simulink model "RWLNN_2m__"  (R2015b)
settings: Solver=ode1  StartTime=0.0  StopTime=t_sim  FixedStep=t_prob  RelTol=1e-3
values from neighbouring files (symbols this model uses):
  ksi = 1    [RWLNN_weights (2).mat]
  lr = 0.01    [RWLNN_weights (2).mat]
  lra = 0.001    [RWLNN_weights (2).mat]
  lrb = 0.001    [RWLNN_weights (2).mat]
  lrin = 0.001    [RWLNN_weights (2).mat]
  T1 = 0.203    [RWLNN_weights (2).mat]
  T2 = 0.203    [RWLNN_weights (2).mat]
  Tc = 0.0012    [RWLNN_weights (2).mat]
  w0 = 40    [RWLNN_weights (2).mat]
  w_init = [0.41  0  0.42; 0  0  -0.04]    [RWLNN_weights (2).mat]
  w_out_init = [-5 0 5]    [RWLNN_weights (2).mat]
undefined symbols (not defined in the file or in its folder): Lz
libraries: neural x3, simulink x1
settings Model: Creator=mateuszzychlewicz  LastModifiedBy=mateuszzychlewicz
settings DataIOCC: LimitDataPoints=off  SaveFormat=Array  TimeSaveName=t  OutputSaveName=y
settings OptimizationCC: EfficientMapNaN2IntZero=off
settings HardwareCC: TargetBitPerLong=64  TargetBitPerPointer=64  TargetLongLongMode=on  TargetIntDivRoundTo=Zero  TargetEndianess=LittleEndian  TargetWordSize=64  TargetHWDeviceType=MATLAB Host  ProdEqTarget=off
settings CodeAppCC: MaxIdLength=128
settings GRTTargetCC: CombineOutputUpdateFcns=off  GRTInterface=on

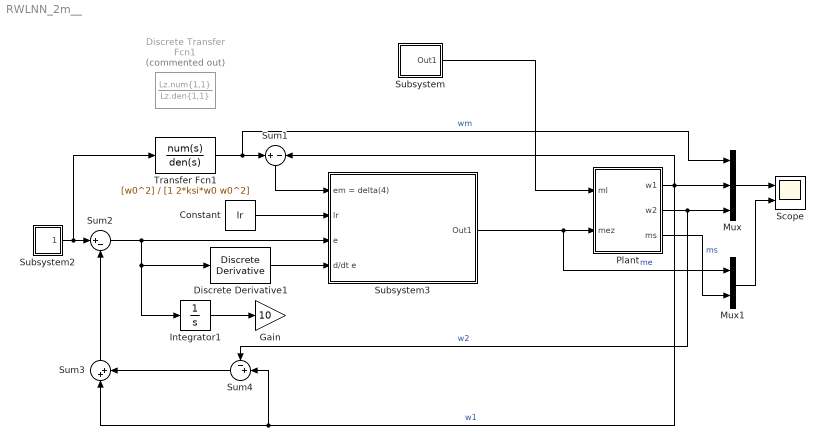
== system RWLNN_2m__ ==
  Constant : Constant  Value=lr
  Discrete Transfer Fcn1 : DiscreteTransferFcn  Commented=on  Numerator=Lz.num{1,1}  Denominator=Lz.den{1,1}
  Discrete Derivative1 : simulink/Discrete/Discrete Derivative  gainval=0.001  ICPrevScaledInput=0.0  InputProcessing=Inherited  OutMin=[]  OutMax=[]  OutDataType=fixdt(1, 16)  OutScaling=2^-10  DoSatur=off
  Gain : Gain  Gain=10
  Integrator1 : Integrator
  Mux : Mux  Inputs=3
  Mux1 : Mux  Inputs=2
  Plant : Subsystem
  Scope : Scope  NumInputPorts=2
  Subsystem : Subsystem
  Subsystem2 : Subsystem
      mask Display: disp('w_{ref}', 'texmode', 'on')
  Subsystem3 : Subsystem
  Sum1 : Sum  Inputs=+-
  Sum2 : Sum  Inputs=|+-
  Sum3 : Sum  Inputs=|++
  Sum4 : Sum  Inputs=-+|
  Transfer Fcn1 : TransferFcn  Numerator=[w0^2]  Denominator=[1 2*ksi*w0 w0^2]
  wires:
  Subsystem2/1(Out1) -> Transfer Fcn1/1, Sum2/1
  Plant/1(w1) -> Sum3/1, Sum4/2, Mux/2, Sum1/2  "w1"
  Sum2/1 -> Discrete Derivative1/1, Integrator1/1, Subsystem3/3(e)
  Transfer Fcn1/1 -> Mux/1, Sum1/1  "wm"
  Sum1/1 -> Subsystem3/1(em = delta(4))
  Plant/2(w2) -> Sum4/1, Mux/3  "w2"
  Mux/1 -> Scope/1
  Plant/3(ms) -> Mux1/2  "ms"
  Mux1/1 -> Scope/2
  Constant/1 -> Subsystem3/2(lr)
  Subsystem/1(Out1) -> Plant/1(ml)
  Integrator1/1 -> Gain/1
  Sum3/1 -> Sum2/2
  Discrete Derivative1/1 -> Subsystem3/4(d/dt e)
  Subsystem3/1(Out1) -> Mux1/1, Plant/2(mez)  "me"
  Sum4/1 -> Sum3/2

== system RWLNN_2m__/Plant ==
  ml : Inport
  mez : Inport  Port=2
  Sum3 : Sum  Inputs=-+|
  Sum4 : Sum  Inputs=-+|
  Sum5 : Sum  Inputs=|+-
  Transfer Fcn1 : TransferFcn  Denominator=[Tc 0]
  Transfer Fcn3 : TransferFcn  Denominator=[T1 0]
  Transfer Fcn4 : TransferFcn  Denominator=[1.5*T2 0]
  w1 : Outport
  w2 : Outport  Port=2
  ms : Outport  Port=3
  wires:
  Sum3/1 -> Transfer Fcn3/1
  mez/1 -> Sum3/2
  ml/1 -> Sum4/1
  Transfer Fcn3/1 -> w1/1, Sum5/1
  Transfer Fcn4/1 -> w2/1, Sum5/2
  Transfer Fcn1/1 -> ms/1, Sum3/1, Sum4/2
  Sum4/1 -> Transfer Fcn4/1
  Sum5/1 -> Transfer Fcn1/1

== system RWLNN_2m__/Subsystem ==
  Step : Step  Time=9  SampleTime=0
  Step1 : Step  Time=11  SampleTime=0
  Sum5 : Sum  Inputs=+-
  Out1 : Outport
  wires:
  Sum5/1 -> Out1/1
  Step/1 -> Sum5/1
  Step1/1 -> Sum5/2

== system RWLNN_2m__/Subsystem2 ==
  Gain : Gain
  Manual Switch : ManualSwitch
  Pulse Generator : DiscretePulseGenerator  PulseType=Time based  Amplitude=0.25  Period=5  PulseWidth=50  PhaseDelay=1
  Pulse Generator1 : DiscretePulseGenerator  PulseType=Time based  Amplitude=0.25  Period=5  PulseWidth=50  PhaseDelay=3.5
  Signal Generator : SignalGenerator  WaveForm=square  Amplitude=0.25  Frequency=0.2
  Sum5 : Sum  Inputs=+-
  Transfer Fcn2 : TransferFcn  Denominator=[0.03 1]
  Out1 : Outport
  wires:
  Sum5/1 -> Manual Switch/2
  Pulse Generator/1 -> Sum5/1
  Pulse Generator1/1 -> Sum5/2
  Signal Generator/1 -> Gain/1
  Gain/1 -> Manual Switch/1
  Manual Switch/1 -> Transfer Fcn2/1
  Transfer Fcn2/1 -> Out1/1

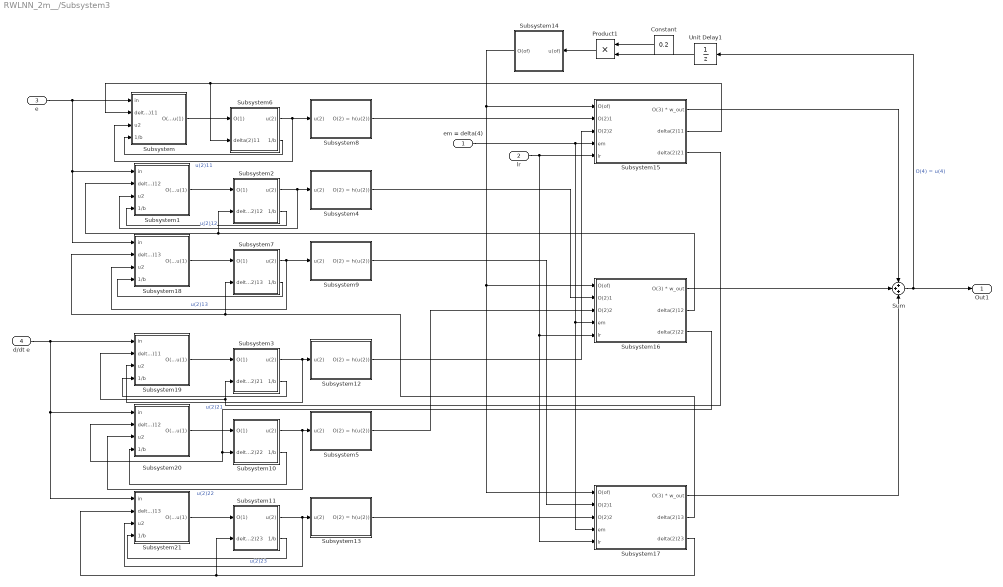
== system RWLNN_2m__/Subsystem3 ==
  em = delta(4) : Inport
  lr : Inport  Port=2
  e : Inport  Port=3
  d/dt e : Inport  Port=4
  Constant : Constant  Value=0.2
  Product1 : Product
  Subsystem : Subsystem
  Subsystem1 : Subsystem
  Subsystem10 : Subsystem
  Subsystem11 : Subsystem
  Subsystem12 : Subsystem
  Subsystem13 : Subsystem
  Subsystem14 : Subsystem
  Subsystem15 : Subsystem
  Subsystem16 : Subsystem
  Subsystem17 : Subsystem
  Subsystem18 : Subsystem
  Subsystem19 : Subsystem
  Subsystem2 : Subsystem
  Subsystem20 : Subsystem
  Subsystem21 : Subsystem
  Subsystem3 : Subsystem
  Subsystem4 : Subsystem
  Subsystem5 : Subsystem
  Subsystem6 : Subsystem
  Subsystem7 : Subsystem
  Subsystem8 : Subsystem
  Subsystem9 : Subsystem
  Sum : Sum  Inputs=+++
  Unit Delay1 : UnitDelay  SampleTime=-1
  Out1 : Outport
  wires:
  Constant/1 -> Product1/1
  Subsystem11/2(1/b) -> Subsystem21/4(1/b)
  Subsystem10/2(1/b) -> Subsystem20/4(1/b)
  Subsystem3/2(1/b) -> Subsystem19/4(1/b)
  d/dt e/1 -> Subsystem19/1(in), Subsystem20/1(in), Subsystem21/1(in)
  Subsystem21/1(O(1) = u(1)) -> Subsystem11/1(O(1))
  Subsystem20/1(O(1) = u(1)) -> Subsystem10/1(O(1))
  Subsystem19/1(O(1) = u(1)) -> Subsystem3/1(O(1))
  Subsystem7/2(1/b) -> Subsystem18/4(1/b)
  Subsystem2/2(1/b) -> Subsystem1/4(1/b)
  Subsystem6/2(1/b) -> Subsystem/4(1/b)
  Subsystem18/1(O(1) = u(1)) -> Subsystem7/1(O(1))
  Subsystem1/1(O(1) = u(1)) -> Subsystem2/1(O(1))
  Subsystem/1(O(1) = u(1)) -> Subsystem6/1(O(1))
  Subsystem17/3(delta(2)23) -> Subsystem11/2(delta(2)23), Subsystem21/2(delta(2)13)
  Subsystem16/3(delta(2)22) -> Subsystem10/2(delta(2)22), Subsystem20/2(delta(2)12)
  Subsystem15/3(delta(2)21) -> Subsystem19/2(delta(2)11), Subsystem3/2(delta(2)21)
  Subsystem17/2(delta(2)13) -> Subsystem18/2(delta(2)13), Subsystem7/2(delta(2)13)
  Subsystem16/2(delta(2)12) -> Subsystem1/2(delta(2)12), Subsystem2/2(delta(2)12)
  Subsystem4/1(O(2) = h(u(2))) -> Subsystem16/2(O(2)1)
  Subsystem5/1(O(2) = h(u(2))) -> Subsystem16/3(O(2)2)
  Subsystem8/1(O(2) = h(u(2))) -> Subsystem15/2(O(2)1)
  Subsystem13/1(O(2) = h(u(2))) -> Subsystem17/3(O(2)2)
  Subsystem12/1(O(2) = h(u(2))) -> Subsystem15/3(O(2)2)
  Subsystem9/1(O(2) = h(u(2))) -> Subsystem17/2(O(2)1)
  Sum/1 -> Unit Delay1/1, Out1/1  "O(4) = u(4)"
  Subsystem15/2(delta(2)11) -> Subsystem6/2(delta(2)11), Subsystem/2(delta(2)11)
  lr/1 -> Subsystem15/5(lr), Subsystem16/5(lr), Subsystem17/5(lr)
  Product1/1 -> Subsystem14/1(u(of))
  Unit Delay1/1 -> Product1/2
  Subsystem7/1(u(2)) -> Subsystem9/1(u(2)), Subsystem18/3(u2)  "u(2)13"
  Subsystem11/1(u(2)) -> Subsystem13/1(u(2)), Subsystem21/3(u2)  "u(2)23"
  Subsystem10/1(u(2)) -> Subsystem5/1(u(2)), Subsystem20/3(u2)  "u(2)22"
  Subsystem3/1(u(2)) -> Subsystem12/1(u(2)), Subsystem19/3(u2)  "u(2)21"
  Subsystem14/1(O(of)) -> Subsystem15/1(O(of)), Subsystem16/1(O(of)), Subsystem17/1(O(of))
  em = delta(4)/1 -> Subsystem15/4(em), Subsystem16/4(em), Subsystem17/4(em)
  Subsystem15/1(O(3) * w_out) -> Sum/1
  e/1 -> Subsystem/1(in), Subsystem1/1(in), Subsystem18/1(in)
  Subsystem2/1(u(2)) -> Subsystem4/1(u(2)), Subsystem1/3(u2)  "u(2)12"
  Subsystem6/1(u(2)) -> Subsystem8/1(u(2)), Subsystem/3(u2)  "u(2)11"
  Subsystem17/1(O(3) * w_out) -> Sum/3
  Subsystem16/1(O(3) * w_out) -> Sum/2

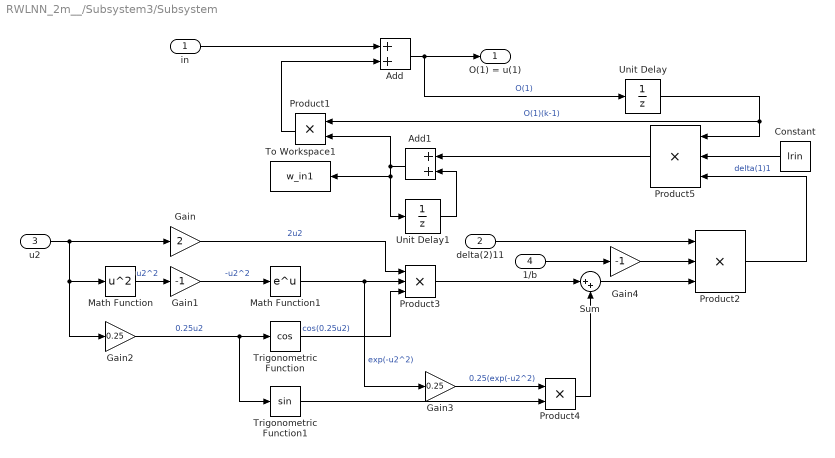
== system RWLNN_2m__/Subsystem3/Subsystem ==
  in : Inport
  delta(2)11 : Inport  Port=2
  u2 : Inport  Port=3
  1/b : Inport  Port=4
  Add : Sum
  Add1 : Sum
  Constant : Constant  Value=lrin
  Gain : Gain  Gain=2
  Gain1 : Gain  Gain=-1
  Gain2 : Gain  Gain=0.25
  Gain3 : Gain  Gain=0.25
  Gain4 : Gain  Gain=-1
  Math Function : Math  Operator=square  SaturateOnIntegerOverflow=on
  Math Function1 : Math  SaturateOnIntegerOverflow=on
  Product1 : Product
  Product2 : Product  Inputs=3
  Product3 : Product  Inputs=3
  Product4 : Product
  Product5 : Product  Inputs=3
  Sum : Sum  Inputs=|++
  To Workspace1 : ToWorkspace  VariableName=w_in1  SampleTime=-1
  Trigonometric Function : Trigonometry  Operator=cos
  Trigonometric Function1 : Trigonometry
  Unit Delay : UnitDelay  SampleTime=-1
  Unit Delay1 : UnitDelay  InitialCondition=w_init(1)  SampleTime=-1
  O(1) = u(1) : Outport
  wires:
  Product1/1 -> Add/2
  Unit Delay1/1 -> Add1/2
  Add1/1 -> Product1/2, Unit Delay1/1, To Workspace1/1
  Product5/1 -> Add1/1
  Constant/1 -> Product5/2
  Product2/1 -> Product5/3  "delta(1)1"
  1/b/1 -> Gain4/1
  Gain4/1 -> Product2/2
  Sum/1 -> Product2/3
  Product4/1 -> Sum/2
  Trigonometric Function1/1 -> Product4/2
  Gain3/1 -> Product4/1  "0.25(exp(-u2^2)"
  Product3/1 -> Sum/1
  Trigonometric Function/1 -> Product3/3  "cos(0.25u2)"
  Gain2/1 -> Trigonometric Function/1, Trigonometric Function1/1  "0.25u2"
  Math Function1/1 -> Product3/2, Gain3/1  "exp(-u2^2)"
  Gain1/1 -> Math Function1/1  "-u2^2"
  Math Function/1 -> Gain1/1  "u2^2"
  Gain/1 -> Product3/1  "2u2"
  u2/1 -> Gain/1, Math Function/1, Gain2/1
  delta(2)11/1 -> Product2/1
  Unit Delay/1 -> Product5/1, Product1/1  "O(1)(k-1)"
  in/1 -> Add/1
  Add/1 -> O(1) = u(1)/1, Unit Delay/1  "O(1)"

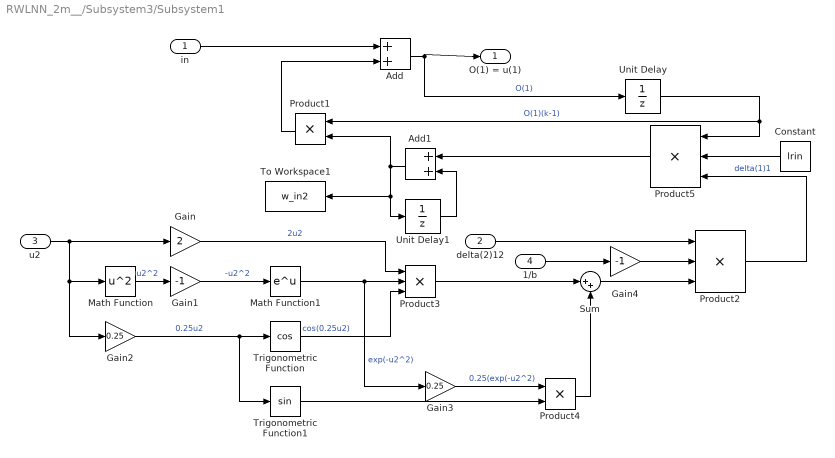
== system RWLNN_2m__/Subsystem3/Subsystem1 ==
  in : Inport
  delta(2)12 : Inport  Port=2
  u2 : Inport  Port=3
  1/b : Inport  Port=4
  Add : Sum
  Add1 : Sum
  Constant : Constant  Value=lrin
  Gain : Gain  Gain=2
  Gain1 : Gain  Gain=-1
  Gain2 : Gain  Gain=0.25
  Gain3 : Gain  Gain=0.25
  Gain4 : Gain  Gain=-1
  Math Function : Math  Operator=square  SaturateOnIntegerOverflow=on
  Math Function1 : Math  SaturateOnIntegerOverflow=on
  Product1 : Product
  Product2 : Product  Inputs=3
  Product3 : Product  Inputs=3
  Product4 : Product
  Product5 : Product  Inputs=3
  Sum : Sum  Inputs=|++
  To Workspace1 : ToWorkspace  VariableName=w_in2  SampleTime=-1
  Trigonometric Function : Trigonometry  Operator=cos
  Trigonometric Function1 : Trigonometry
  Unit Delay : UnitDelay  SampleTime=-1
  Unit Delay1 : UnitDelay  InitialCondition=w_init(2)  SampleTime=-1
  O(1) = u(1) : Outport
  wires:
  Add1/1 -> Unit Delay1/1, To Workspace1/1, Product1/2
  Add/1 -> Unit Delay/1, O(1) = u(1)/1  "O(1)"
  in/1 -> Add/1
  Unit Delay/1 -> Product1/1, Product5/1  "O(1)(k-1)"
  delta(2)12/1 -> Product2/1
  u2/1 -> Gain2/1, Math Function/1, Gain/1
  Gain/1 -> Product3/1  "2u2"
  Math Function/1 -> Gain1/1  "u2^2"
  Gain1/1 -> Math Function1/1  "-u2^2"
  Math Function1/1 -> Gain3/1, Product3/2  "exp(-u2^2)"
  Gain2/1 -> Trigonometric Function1/1, Trigonometric Function/1  "0.25u2"
  Trigonometric Function/1 -> Product3/3  "cos(0.25u2)"
  Product3/1 -> Sum/1
  Gain3/1 -> Product4/1  "0.25(exp(-u2^2)"
  Trigonometric Function1/1 -> Product4/2
  Product4/1 -> Sum/2
  Sum/1 -> Product2/3
  Gain4/1 -> Product2/2
  1/b/1 -> Gain4/1
  Product2/1 -> Product5/3  "delta(1)1"
  Constant/1 -> Product5/2
  Product5/1 -> Add1/1
  Unit Delay1/1 -> Add1/2
  Product1/1 -> Add/2

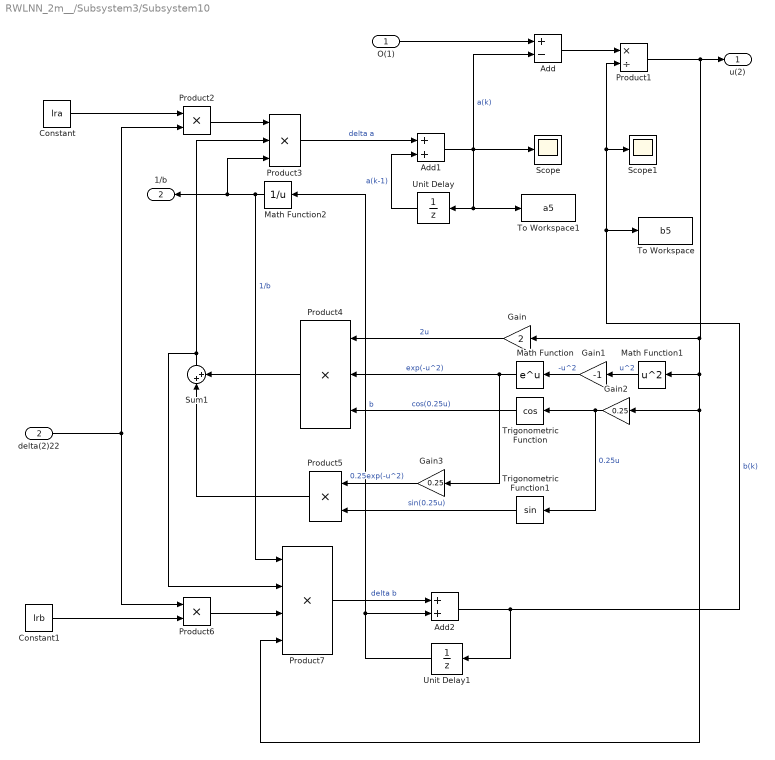
== system RWLNN_2m__/Subsystem3/Subsystem10 ==
  O(1) : Inport
  delta(2)22 : Inport  Port=2
  Add : Sum  Inputs=+-
  Add1 : Sum  Inputs=2
  Add2 : Sum  Inputs=2
  Constant : Constant  Value=lra
  Constant1 : Constant  Value=lrb
  Gain : Gain  Gain=2
  Gain1 : Gain  Gain=-1
  Gain2 : Gain  Gain=0.25
  Gain3 : Gain  Gain=0.25
  Math Function : Math  SaturateOnIntegerOverflow=on
  Math Function1 : Math  Operator=square  SaturateOnIntegerOverflow=on
  Math Function2 : Math  Operator=reciprocal  SaturateOnIntegerOverflow=on
  Product1 : Product  Inputs=*/
  Product2 : Product
  Product3 : Product  Inputs=3
  Product4 : Product  Inputs=3
  Product5 : Product
  Product6 : Product
  Product7 : Product  Inputs=4
  Scope : Scope
  Scope1 : Scope
  Sum1 : Sum  Inputs=|++
  To Workspace : ToWorkspace  VariableName=b5  SampleTime=-1
  To Workspace1 : ToWorkspace  VariableName=a5  SampleTime=-1
  Trigonometric Function : Trigonometry  Operator=cos
  Trigonometric Function1 : Trigonometry
  Unit Delay : UnitDelay  SampleTime=-1
  Unit Delay1 : UnitDelay  InitialCondition=1  SampleTime=-1
  u(2) : Outport
  1/b : Outport  Port=2
  wires:
  Add2/1 -> Unit Delay1/1, Product1/2, Scope1/1, To Workspace/1  "b(k)"
  Product7/1 -> Add2/1  "delta b"
  Product6/1 -> Product7/3
  Constant1/1 -> Product6/2
  delta(2)22/1 -> Product2/2, Product6/1
  Constant/1 -> Product2/1
  Unit Delay/1 -> Add1/2  "a(k-1)"
  Add1/1 -> Add/2, To Workspace1/1, Unit Delay/1, Scope/1  "a(k)"
  Product3/1 -> Add1/1  "delta a"
  Unit Delay1/1 -> Math Function2/1, Add2/2  "b"
  Math Function2/1 -> Product3/3, 1/b/1, Product7/1  "1/b"
  Sum1/1 -> Product7/2, Product3/2
  Product5/1 -> Sum1/1
  Trigonometric Function1/1 -> Product5/2  "sin(0.25u)"
  Gain3/1 -> Product5/1  "0.25exp(-u^2)"
  Product4/1 -> Sum1/2
  Trigonometric Function/1 -> Product4/3  "cos(0.25u)"
  Gain2/1 -> Trigonometric Function1/1, Trigonometric Function/1  "0.25u"
  Math Function/1 -> Gain3/1, Product4/2  "exp(-u^2)"
  Gain1/1 -> Math Function/1  "-u^2"
  Math Function1/1 -> Gain1/1  "u^2"
  Gain/1 -> Product4/1  "2u"
  Product1/1 -> u(2)/1, Gain/1, Math Function1/1, Gain2/1, Product7/4
  Product2/1 -> Product3/1
  Add/1 -> Product1/1
  O(1)/1 -> Add/1

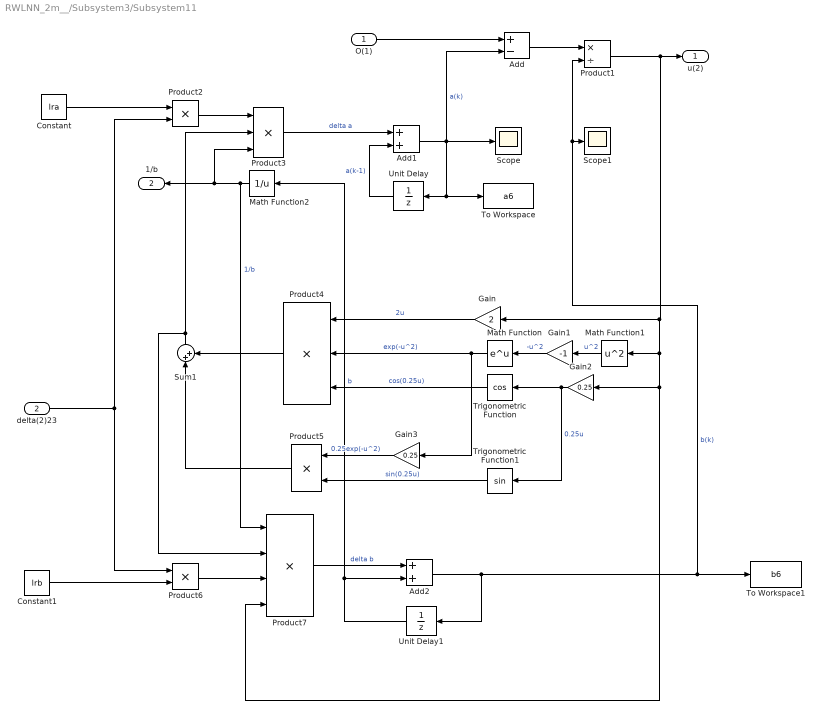
== system RWLNN_2m__/Subsystem3/Subsystem11 ==
  O(1) : Inport
  delta(2)23 : Inport  Port=2
  Add : Sum  Inputs=+-
  Add1 : Sum  Inputs=2
  Add2 : Sum  Inputs=2
  Constant : Constant  Value=lra
  Constant1 : Constant  Value=lrb
  Gain : Gain  Gain=2
  Gain1 : Gain  Gain=-1
  Gain2 : Gain  Gain=0.25
  Gain3 : Gain  Gain=0.25
  Math Function : Math  SaturateOnIntegerOverflow=on
  Math Function1 : Math  Operator=square  SaturateOnIntegerOverflow=on
  Math Function2 : Math  Operator=reciprocal  SaturateOnIntegerOverflow=on
  Product1 : Product  Inputs=*/
  Product2 : Product
  Product3 : Product  Inputs=3
  Product4 : Product  Inputs=3
  Product5 : Product
  Product6 : Product
  Product7 : Product  Inputs=4
  Scope : Scope
  Scope1 : Scope
  Sum1 : Sum  Inputs=|++
  To Workspace : ToWorkspace  VariableName=a6  SampleTime=-1
  To Workspace1 : ToWorkspace  VariableName=b6  SampleTime=-1
  Trigonometric Function : Trigonometry  Operator=cos
  Trigonometric Function1 : Trigonometry
  Unit Delay : UnitDelay  InitialCondition=0.26  SampleTime=-1
  Unit Delay1 : UnitDelay  InitialCondition=1.13  SampleTime=-1
  u(2) : Outport
  1/b : Outport  Port=2
  wires:
  O(1)/1 -> Add/1
  Add/1 -> Product1/1
  Product2/1 -> Product3/1
  Product1/1 -> Product7/4, Gain2/1, Math Function1/1, Gain/1, u(2)/1
  Gain/1 -> Product4/1  "2u"
  Math Function1/1 -> Gain1/1  "u^2"
  Gain1/1 -> Math Function/1  "-u^2"
  Math Function/1 -> Product4/2, Gain3/1  "exp(-u^2)"
  Gain2/1 -> Trigonometric Function/1, Trigonometric Function1/1  "0.25u"
  Trigonometric Function/1 -> Product4/3  "cos(0.25u)"
  Product4/1 -> Sum1/2
  Gain3/1 -> Product5/1  "0.25exp(-u^2)"
  Trigonometric Function1/1 -> Product5/2  "sin(0.25u)"
  Product5/1 -> Sum1/1
  Sum1/1 -> Product3/2, Product7/2
  Math Function2/1 -> Product7/1, Product3/3, 1/b/1  "1/b"
  Unit Delay1/1 -> Add2/2, Math Function2/1  "b"
  Product3/1 -> Add1/1  "delta a"
  Add1/1 -> To Workspace/1, Unit Delay/1, Add/2, Scope/1  "a(k)"
  Unit Delay/1 -> Add1/2  "a(k-1)"
  Constant/1 -> Product2/1
  delta(2)23/1 -> Product6/1, Product2/2
  Constant1/1 -> Product6/2
  Product6/1 -> Product7/3
  Product7/1 -> Add2/1  "delta b"
  Add2/1 -> Product1/2, Scope1/1, To Workspace1/1, Unit Delay1/1  "b(k)"

== system RWLNN_2m__/Subsystem3/Subsystem12 ==
  u(2) : Inport
  Gain : Gain  Gain=0.25
  Gain1 : Gain  Gain=-1
  Math Function : Math  SaturateOnIntegerOverflow=on
  Product1 : Product
  Product2 : Product
  Trigonometric Function : Trigonometry  Operator=cos
  O(2) = h(u(2)) : Outport
  wires:
  Product2/1 -> Gain1/1  "u(2) ^ 2"
  Product1/1 -> O(2) = h(u(2))/1
  Gain/1 -> Trigonometric Function/1  "0.25 * u(2)"
  Gain1/1 -> Math Function/1  "-(u(2) ^ 2)"
  Trigonometric Function/1 -> Product1/1
  u(2)/1 -> Product2/1, Product2/2, Gain/1
  Math Function/1 -> Product1/2

== system RWLNN_2m__/Subsystem3/Subsystem13 ==
  u(2) : Inport
  Gain : Gain  Gain=0.25
  Gain1 : Gain  Gain=-1
  Math Function : Math  SaturateOnIntegerOverflow=on
  Product1 : Product
  Product2 : Product
  Trigonometric Function : Trigonometry  Operator=cos
  O(2) = h(u(2)) : Outport
  wires:
  Math Function/1 -> Product1/2
  u(2)/1 -> Gain/1, Product2/2, Product2/1
  Trigonometric Function/1 -> Product1/1
  Gain1/1 -> Math Function/1  "-(u(2) ^ 2)"
  Gain/1 -> Trigonometric Function/1  "0.25 * u(2)"
  Product1/1 -> O(2) = h(u(2))/1
  Product2/1 -> Gain1/1  "u(2) ^ 2"

== system RWLNN_2m__/Subsystem3/Subsystem14 ==
  u(of) : Inport
  Gain1 : Gain  Gain=-1
  Math Function : Math  SaturateOnIntegerOverflow=on
  Product2 : Product
  O(of) : Outport
  wires:
  Math Function/1 -> O(of)/1
  u(of)/1 -> Product2/1, Product2/2
  Gain1/1 -> Math Function/1  "-(u(of) ^ 2)"
  Product2/1 -> Gain1/1  "u(of) ^ 2"

== system RWLNN_2m__/Subsystem3/Subsystem15 ==
  O(of) : Inport
  O(2)1 : Inport  Port=2
  O(2)2 : Inport  Port=3
  em : Inport  Port=4
  lr : Inport  Port=5
  Add : Sum
  Manual Switch : ManualSwitch  CurrentSetting=0
  Product : Product  Inputs=4
  Product{1,3,5..6} (4 alike) : Product
  Product2 : Product  Inputs=3
  Product4 : Product  Inputs=3
  To Workspace : ToWorkspace  VariableName=w_out1  SampleTime=-1
  Unit Delay : UnitDelay  SampleTime=-1
  Unit Delay1 : UnitDelay  InitialCondition=w_out_init(1)  SampleTime=-1
  logsig : neural/Transfer Functions/logsig
  O(3) * w_out : Outport
  delta(2)11 : Outport  Port=2
  delta(2)21 : Outport  Port=3
  wires:
  Product5/1 -> delta(2)11/1
  Product6/1 -> delta(2)21/1
  Product4/1 -> Product5/2, Product6/2
  Product3/1 -> Product4/1
  Manual Switch/1 -> Product3/2
  Unit Delay1/1 -> Manual Switch/1, Add/2  "w_out(k - 1)"
  Add/1 -> Unit Delay1/1, Manual Switch/2, To Workspace/1, Product1/2  "w_out(k)"
  Product2/1 -> Add/1  "delta w_out"
  em/1 -> Product2/2, Product3/1
  lr/1 -> Product2/3
  Product1/1 -> O(3) * w_out/1
  O(of)/1 -> Product/1, Product4/2
  O(2)2/1 -> Product/3, Product6/1
  Product/1 -> Unit Delay/1, Product1/1, Product2/1
  Unit Delay/1 -> logsig/1
  logsig/1 -> Product4/3, Product/4
  O(2)1/1 -> Product5/1, Product/2

== system RWLNN_2m__/Subsystem3/Subsystem16 ==
  O(of) : Inport
  O(2)1 : Inport  Port=2
  O(2)2 : Inport  Port=3
  em : Inport  Port=4
  lr : Inport  Port=5
  Add : Sum
  Manual Switch : ManualSwitch  CurrentSetting=0
  Product : Product  Inputs=4
  Product{1,3,5..6} (4 alike) : Product
  Product2 : Product  Inputs=3
  Product4 : Product  Inputs=3
  To Workspace : ToWorkspace  VariableName=w_out2  SampleTime=-1
  Unit Delay : UnitDelay  SampleTime=-1
  Unit Delay1 : UnitDelay  InitialCondition=w_out_init(2)  SampleTime=-1
  logsig : neural/Transfer Functions/logsig
  O(3) * w_out : Outport
  delta(2)12 : Outport  Port=2
  delta(2)22 : Outport  Port=3
  wires:
  O(2)1/1 -> Product/2, Product5/1
  logsig/1 -> Product/4, Product4/3
  Unit Delay/1 -> logsig/1
  Product/1 -> Product2/1, Product1/1, Unit Delay/1
  O(2)2/1 -> Product6/1, Product/3
  O(of)/1 -> Product4/2, Product/1
  Product1/1 -> O(3) * w_out/1
  lr/1 -> Product2/3
  em/1 -> Product3/1, Product2/2
  Product2/1 -> Add/1  "delta w_out"
  Add/1 -> Product1/2, Manual Switch/2, To Workspace/1, Unit Delay1/1  "w_out(k)"
  Unit Delay1/1 -> Add/2, Manual Switch/1  "w_out(k - 1)"
  Manual Switch/1 -> Product3/2
  Product3/1 -> Product4/1
  Product4/1 -> Product6/2, Product5/2
  Product6/1 -> delta(2)22/1
  Product5/1 -> delta(2)12/1

== system RWLNN_2m__/Subsystem3/Subsystem17 ==
  O(of) : Inport
  O(2)1 : Inport  Port=2
  O(2)2 : Inport  Port=3
  em : Inport  Port=4
  lr : Inport  Port=5
  Add : Sum
  Manual Switch : ManualSwitch  CurrentSetting=0
  Product : Product  Inputs=4
  Product{1,3,5..6} (4 alike) : Product
  Product2 : Product  Inputs=3
  Product4 : Product  Inputs=3
  To Workspace : ToWorkspace  VariableName=w_out3  SampleTime=-1
  Unit Delay : UnitDelay  SampleTime=-1
  Unit Delay1 : UnitDelay  InitialCondition=w_out_init(3)  SampleTime=-1
  logsig : neural/Transfer Functions/logsig
  O(3) * w_out : Outport
  delta(2)13 : Outport  Port=2
  delta(2)23 : Outport  Port=3
  wires:
  Product5/1 -> delta(2)13/1
  Product6/1 -> delta(2)23/1
  Product4/1 -> Product5/2, Product6/2
  Product3/1 -> Product4/1
  Manual Switch/1 -> Product3/2
  Unit Delay1/1 -> Manual Switch/1, Add/2  "w_out(k - 1)"
  Add/1 -> Manual Switch/2, To Workspace/1, Unit Delay1/1, Product1/2  "w_out(k)"
  Product2/1 -> Add/1  "delta w_out"
  em/1 -> Product2/2, Product3/1
  lr/1 -> Product2/3
  Product1/1 -> O(3) * w_out/1
  O(of)/1 -> Product/1, Product4/2
  O(2)2/1 -> Product/3, Product6/1
  Product/1 -> Unit Delay/1, Product1/1, Product2/1
  Unit Delay/1 -> logsig/1
  logsig/1 -> Product4/3, Product/4
  O(2)1/1 -> Product5/1, Product/2

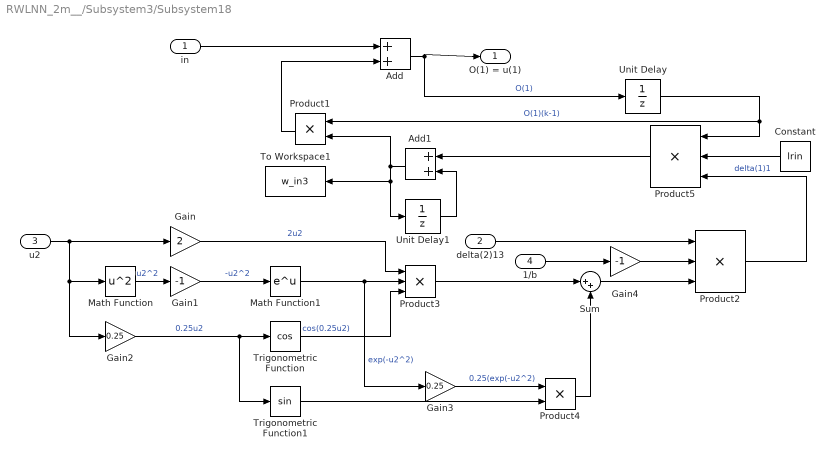
== system RWLNN_2m__/Subsystem3/Subsystem18 ==
  in : Inport
  delta(2)13 : Inport  Port=2
  u2 : Inport  Port=3
  1/b : Inport  Port=4
  Add : Sum
  Add1 : Sum
  Constant : Constant  Value=lrin
  Gain : Gain  Gain=2
  Gain1 : Gain  Gain=-1
  Gain2 : Gain  Gain=0.25
  Gain3 : Gain  Gain=0.25
  Gain4 : Gain  Gain=-1
  Math Function : Math  Operator=square  SaturateOnIntegerOverflow=on
  Math Function1 : Math  SaturateOnIntegerOverflow=on
  Product1 : Product
  Product2 : Product  Inputs=3
  Product3 : Product  Inputs=3
  Product4 : Product
  Product5 : Product  Inputs=3
  Sum : Sum  Inputs=|++
  To Workspace1 : ToWorkspace  VariableName=w_in3  SampleTime=-1
  Trigonometric Function : Trigonometry  Operator=cos
  Trigonometric Function1 : Trigonometry
  Unit Delay : UnitDelay  SampleTime=-1
  Unit Delay1 : UnitDelay  InitialCondition=w_init(3)  SampleTime=-1
  O(1) = u(1) : Outport
  wires:
  Product1/1 -> Add/2
  Unit Delay1/1 -> Add1/2
  Add1/1 -> Product1/2, Unit Delay1/1, To Workspace1/1
  Product5/1 -> Add1/1
  Constant/1 -> Product5/2
  Product2/1 -> Product5/3  "delta(1)1"
  1/b/1 -> Gain4/1
  Gain4/1 -> Product2/2
  Sum/1 -> Product2/3
  Product4/1 -> Sum/2
  Trigonometric Function1/1 -> Product4/2
  Gain3/1 -> Product4/1  "0.25(exp(-u2^2)"
  Product3/1 -> Sum/1
  Trigonometric Function/1 -> Product3/3  "cos(0.25u2)"
  Gain2/1 -> Trigonometric Function/1, Trigonometric Function1/1  "0.25u2"
  Math Function1/1 -> Product3/2, Gain3/1  "exp(-u2^2)"
  Gain1/1 -> Math Function1/1  "-u2^2"
  Math Function/1 -> Gain1/1  "u2^2"
  Gain/1 -> Product3/1  "2u2"
  u2/1 -> Gain/1, Math Function/1, Gain2/1
  delta(2)13/1 -> Product2/1
  Unit Delay/1 -> Product5/1, Product1/1  "O(1)(k-1)"
  in/1 -> Add/1
  Add/1 -> O(1) = u(1)/1, Unit Delay/1  "O(1)"

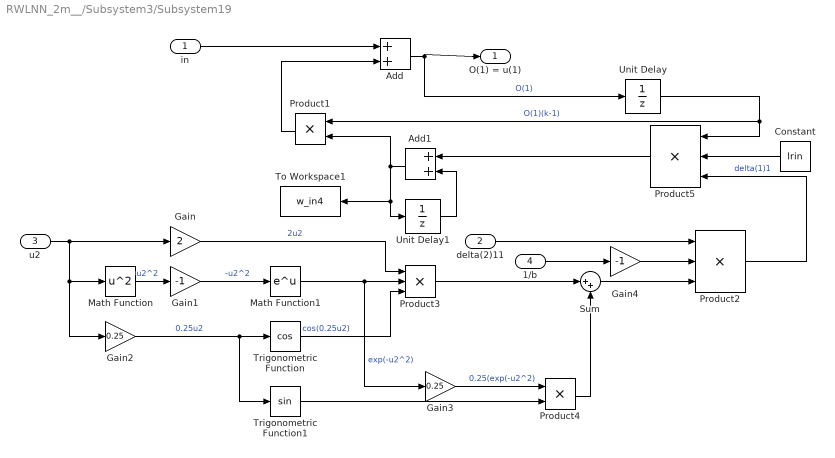
== system RWLNN_2m__/Subsystem3/Subsystem19 ==
  in : Inport
  delta(2)11 : Inport  Port=2
  u2 : Inport  Port=3
  1/b : Inport  Port=4
  Add : Sum
  Add1 : Sum
  Constant : Constant  Value=lrin
  Gain : Gain  Gain=2
  Gain1 : Gain  Gain=-1
  Gain2 : Gain  Gain=0.25
  Gain3 : Gain  Gain=0.25
  Gain4 : Gain  Gain=-1
  Math Function : Math  Operator=square  SaturateOnIntegerOverflow=on
  Math Function1 : Math  SaturateOnIntegerOverflow=on
  Product1 : Product
  Product2 : Product  Inputs=3
  Product3 : Product  Inputs=3
  Product4 : Product
  Product5 : Product  Inputs=3
  Sum : Sum  Inputs=|++
  To Workspace1 : ToWorkspace  VariableName=w_in4  SampleTime=-1
  Trigonometric Function : Trigonometry  Operator=cos
  Trigonometric Function1 : Trigonometry
  Unit Delay : UnitDelay  SampleTime=-1
  Unit Delay1 : UnitDelay  InitialCondition=w_init(4)  SampleTime=-1
  O(1) = u(1) : Outport
  wires:
  Add/1 -> Unit Delay/1, O(1) = u(1)/1  "O(1)"
  in/1 -> Add/1
  Unit Delay/1 -> Product1/1, Product5/1  "O(1)(k-1)"
  delta(2)11/1 -> Product2/1
  u2/1 -> Gain2/1, Math Function/1, Gain/1
  Gain/1 -> Product3/1  "2u2"
  Math Function/1 -> Gain1/1  "u2^2"
  Gain1/1 -> Math Function1/1  "-u2^2"
  Math Function1/1 -> Gain3/1, Product3/2  "exp(-u2^2)"
  Gain2/1 -> Trigonometric Function1/1, Trigonometric Function/1  "0.25u2"
  Trigonometric Function/1 -> Product3/3  "cos(0.25u2)"
  Product3/1 -> Sum/1
  Gain3/1 -> Product4/1  "0.25(exp(-u2^2)"
  Trigonometric Function1/1 -> Product4/2
  Product4/1 -> Sum/2
  Sum/1 -> Product2/3
  Gain4/1 -> Product2/2
  1/b/1 -> Gain4/1
  Product2/1 -> Product5/3  "delta(1)1"
  Constant/1 -> Product5/2
  Product5/1 -> Add1/1
  Add1/1 -> Unit Delay1/1, To Workspace1/1, Product1/2
  Unit Delay1/1 -> Add1/2
  Product1/1 -> Add/2

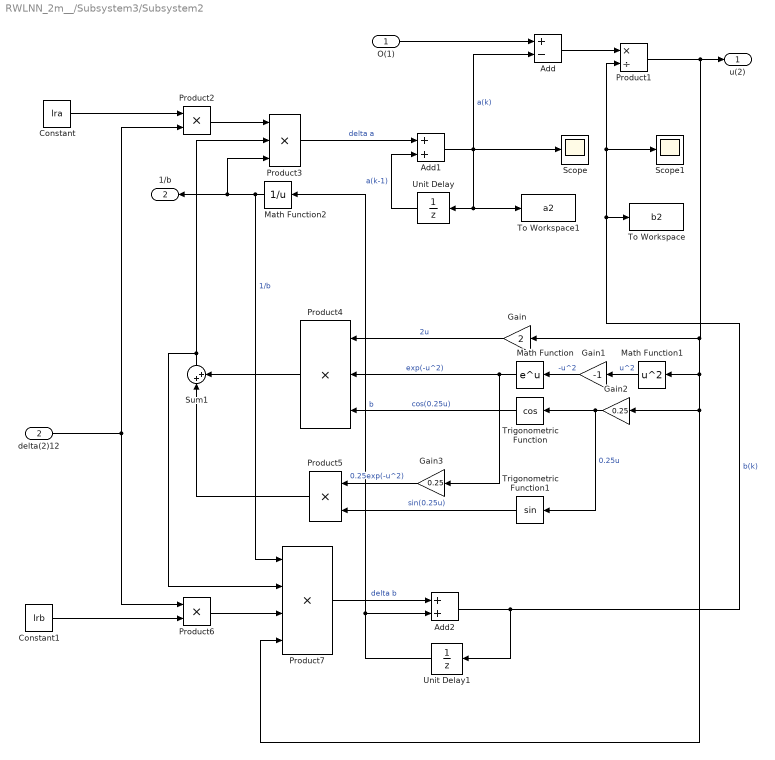
== system RWLNN_2m__/Subsystem3/Subsystem2 ==
  O(1) : Inport
  delta(2)12 : Inport  Port=2
  Add : Sum  Inputs=+-
  Add1 : Sum  Inputs=2
  Add2 : Sum  Inputs=2
  Constant : Constant  Value=lra
  Constant1 : Constant  Value=lrb
  Gain : Gain  Gain=2
  Gain1 : Gain  Gain=-1
  Gain2 : Gain  Gain=0.25
  Gain3 : Gain  Gain=0.25
  Math Function : Math  SaturateOnIntegerOverflow=on
  Math Function1 : Math  Operator=square  SaturateOnIntegerOverflow=on
  Math Function2 : Math  Operator=reciprocal  SaturateOnIntegerOverflow=on
  Product1 : Product  Inputs=*/
  Product2 : Product
  Product3 : Product  Inputs=3
  Product4 : Product  Inputs=3
  Product5 : Product
  Product6 : Product
  Product7 : Product  Inputs=4
  Scope : Scope
  Scope1 : Scope
  Sum1 : Sum  Inputs=|++
  To Workspace : ToWorkspace  VariableName=b2  SampleTime=-1
  To Workspace1 : ToWorkspace  VariableName=a2  SampleTime=-1
  Trigonometric Function : Trigonometry  Operator=cos
  Trigonometric Function1 : Trigonometry
  Unit Delay : UnitDelay  SampleTime=-1
  Unit Delay1 : UnitDelay  InitialCondition=1.02  SampleTime=-1
  u(2) : Outport
  1/b : Outport  Port=2
  wires:
  O(1)/1 -> Add/1
  Add/1 -> Product1/1
  Product2/1 -> Product3/1
  Product1/1 -> Product7/4, Gain2/1, Math Function1/1, Gain/1, u(2)/1
  Gain/1 -> Product4/1  "2u"
  Math Function1/1 -> Gain1/1  "u^2"
  Gain1/1 -> Math Function/1  "-u^2"
  Math Function/1 -> Product4/2, Gain3/1  "exp(-u^2)"
  Gain2/1 -> Trigonometric Function/1, Trigonometric Function1/1  "0.25u"
  Trigonometric Function/1 -> Product4/3  "cos(0.25u)"
  Product4/1 -> Sum1/2
  Gain3/1 -> Product5/1  "0.25exp(-u^2)"
  Trigonometric Function1/1 -> Product5/2  "sin(0.25u)"
  Product5/1 -> Sum1/1
  Sum1/1 -> Product3/2, Product7/2
  Math Function2/1 -> Product7/1, Product3/3, 1/b/1  "1/b"
  Unit Delay1/1 -> Add2/2, Math Function2/1  "b"
  Product3/1 -> Add1/1  "delta a"
  Add1/1 -> Unit Delay/1, To Workspace1/1, Add/2, Scope/1  "a(k)"
  Unit Delay/1 -> Add1/2  "a(k-1)"
  Constant/1 -> Product2/1
  delta(2)12/1 -> Product6/1, Product2/2
  Constant1/1 -> Product6/2
  Product6/1 -> Product7/3
  Product7/1 -> Add2/1  "delta b"
  Add2/1 -> Product1/2, Scope1/1, To Workspace/1, Unit Delay1/1  "b(k)"

== system RWLNN_2m__/Subsystem3/Subsystem20 ==
  in : Inport
  delta(2)12 : Inport  Port=2
  u2 : Inport  Port=3
  1/b : Inport  Port=4
  Add : Sum
  Add1 : Sum
  Constant : Constant  Value=lrin
  Gain : Gain  Gain=2
  Gain1 : Gain  Gain=-1
  Gain2 : Gain  Gain=0.25
  Gain3 : Gain  Gain=0.25
  Gain4 : Gain  Gain=-1
  Math Function : Math  Operator=square  SaturateOnIntegerOverflow=on
  Math Function1 : Math  SaturateOnIntegerOverflow=on
  Product1 : Product
  Product2 : Product  Inputs=3
  Product3 : Product  Inputs=3
  Product4 : Product
  Product5 : Product  Inputs=3
  Sum : Sum  Inputs=|++
  To Workspace1 : ToWorkspace  VariableName=w_in5  SampleTime=-1
  Trigonometric Function : Trigonometry  Operator=cos
  Trigonometric Function1 : Trigonometry
  Unit Delay : UnitDelay  SampleTime=-1
  Unit Delay1 : UnitDelay  InitialCondition=w_init(5)  SampleTime=-1
  O(1) = u(1) : Outport
  wires:
  Product1/1 -> Add/2
  Unit Delay1/1 -> Add1/2
  Add1/1 -> Product1/2, Unit Delay1/1, To Workspace1/1
  Product5/1 -> Add1/1
  Constant/1 -> Product5/2
  Product2/1 -> Product5/3  "delta(1)1"
  1/b/1 -> Gain4/1
  Gain4/1 -> Product2/2
  Sum/1 -> Product2/3
  Product4/1 -> Sum/2
  Trigonometric Function1/1 -> Product4/2
  Gain3/1 -> Product4/1  "0.25(exp(-u2^2)"
  Product3/1 -> Sum/1
  Trigonometric Function/1 -> Product3/3  "cos(0.25u2)"
  Gain2/1 -> Trigonometric Function/1, Trigonometric Function1/1  "0.25u2"
  Math Function1/1 -> Product3/2, Gain3/1  "exp(-u2^2)"
  Gain1/1 -> Math Function1/1  "-u2^2"
  Math Function/1 -> Gain1/1  "u2^2"
  Gain/1 -> Product3/1  "2u2"
  u2/1 -> Gain/1, Math Function/1, Gain2/1
  delta(2)12/1 -> Product2/1
  Unit Delay/1 -> Product5/1, Product1/1  "O(1)(k-1)"
  in/1 -> Add/1
  Add/1 -> O(1) = u(1)/1, Unit Delay/1  "O(1)"

== system RWLNN_2m__/Subsystem3/Subsystem21 ==
  in : Inport
  delta(2)13 : Inport  Port=2
  u2 : Inport  Port=3
  1/b : Inport  Port=4
  Add : Sum
  Add1 : Sum
  Constant : Constant  Value=lrin
  Gain : Gain  Gain=2
  Gain1 : Gain  Gain=-1
  Gain2 : Gain  Gain=0.25
  Gain3 : Gain  Gain=0.25
  Gain4 : Gain  Gain=-1
  Math Function : Math  Operator=square  SaturateOnIntegerOverflow=on
  Math Function1 : Math  SaturateOnIntegerOverflow=on
  Product1 : Product
  Product2 : Product  Inputs=3
  Product3 : Product  Inputs=3
  Product4 : Product
  Product5 : Product  Inputs=3
  Sum : Sum  Inputs=|++
  To Workspace1 : ToWorkspace  VariableName=w_in6  SampleTime=-1
  Trigonometric Function : Trigonometry  Operator=cos
  Trigonometric Function1 : Trigonometry
  Unit Delay : UnitDelay  SampleTime=-1
  Unit Delay1 : UnitDelay  InitialCondition=w_init(6)  SampleTime=-1
  O(1) = u(1) : Outport
  wires:
  Add/1 -> Unit Delay/1, O(1) = u(1)/1  "O(1)"
  in/1 -> Add/1
  Unit Delay/1 -> Product1/1, Product5/1  "O(1)(k-1)"
  delta(2)13/1 -> Product2/1
  u2/1 -> Gain2/1, Math Function/1, Gain/1
  Gain/1 -> Product3/1  "2u2"
  Math Function/1 -> Gain1/1  "u2^2"
  Gain1/1 -> Math Function1/1  "-u2^2"
  Math Function1/1 -> Gain3/1, Product3/2  "exp(-u2^2)"
  Gain2/1 -> Trigonometric Function1/1, Trigonometric Function/1  "0.25u2"
  Trigonometric Function/1 -> Product3/3  "cos(0.25u2)"
  Product3/1 -> Sum/1
  Gain3/1 -> Product4/1  "0.25(exp(-u2^2)"
  Trigonometric Function1/1 -> Product4/2
  Product4/1 -> Sum/2
  Sum/1 -> Product2/3
  Gain4/1 -> Product2/2
  1/b/1 -> Gain4/1
  Product2/1 -> Product5/3  "delta(1)1"
  Constant/1 -> Product5/2
  Product5/1 -> Add1/1
  Add1/1 -> Unit Delay1/1, To Workspace1/1, Product1/2
  Unit Delay1/1 -> Add1/2
  Product1/1 -> Add/2

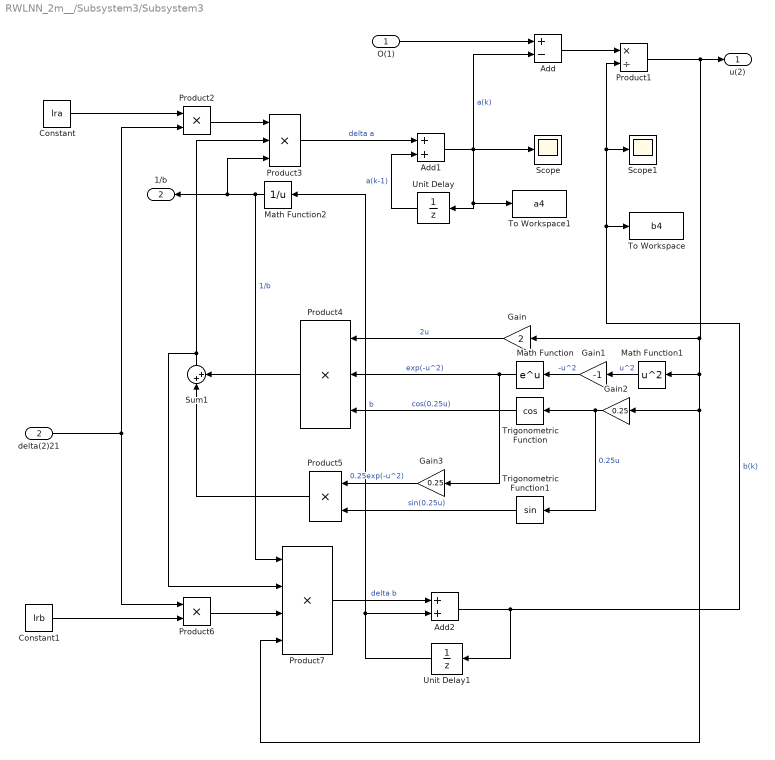
== system RWLNN_2m__/Subsystem3/Subsystem3 ==
  O(1) : Inport
  delta(2)21 : Inport  Port=2
  Add : Sum  Inputs=+-
  Add1 : Sum  Inputs=2
  Add2 : Sum  Inputs=2
  Constant : Constant  Value=lra
  Constant1 : Constant  Value=lrb
  Gain : Gain  Gain=2
  Gain1 : Gain  Gain=-1
  Gain2 : Gain  Gain=0.25
  Gain3 : Gain  Gain=0.25
  Math Function : Math  SaturateOnIntegerOverflow=on
  Math Function1 : Math  Operator=square  SaturateOnIntegerOverflow=on
  Math Function2 : Math  Operator=reciprocal  SaturateOnIntegerOverflow=on
  Product1 : Product  Inputs=*/
  Product2 : Product
  Product3 : Product  Inputs=3
  Product4 : Product  Inputs=3
  Product5 : Product
  Product6 : Product
  Product7 : Product  Inputs=4
  Scope : Scope
  Scope1 : Scope
  Sum1 : Sum  Inputs=|++
  To Workspace : ToWorkspace  VariableName=b4  SampleTime=-1
  To Workspace1 : ToWorkspace  VariableName=a4  SampleTime=-1
  Trigonometric Function : Trigonometry  Operator=cos
  Trigonometric Function1 : Trigonometry
  Unit Delay : UnitDelay  InitialCondition=-0.26  SampleTime=-1
  Unit Delay1 : UnitDelay  InitialCondition=1.12  SampleTime=-1
  u(2) : Outport
  1/b : Outport  Port=2
  wires:
  O(1)/1 -> Add/1
  Add/1 -> Product1/1
  Product2/1 -> Product3/1
  Product1/1 -> Product7/4, Gain2/1, Math Function1/1, Gain/1, u(2)/1
  Gain/1 -> Product4/1  "2u"
  Math Function1/1 -> Gain1/1  "u^2"
  Gain1/1 -> Math Function/1  "-u^2"
  Math Function/1 -> Product4/2, Gain3/1  "exp(-u^2)"
  Gain2/1 -> Trigonometric Function/1, Trigonometric Function1/1  "0.25u"
  Trigonometric Function/1 -> Product4/3  "cos(0.25u)"
  Product4/1 -> Sum1/2
  Gain3/1 -> Product5/1  "0.25exp(-u^2)"
  Trigonometric Function1/1 -> Product5/2  "sin(0.25u)"
  Product5/1 -> Sum1/1
  Sum1/1 -> Product3/2, Product7/2
  Math Function2/1 -> Product7/1, Product3/3, 1/b/1  "1/b"
  Unit Delay1/1 -> Add2/2, Math Function2/1  "b"
  Product3/1 -> Add1/1  "delta a"
  Add1/1 -> Unit Delay/1, To Workspace1/1, Add/2, Scope/1  "a(k)"
  Unit Delay/1 -> Add1/2  "a(k-1)"
  Constant/1 -> Product2/1
  delta(2)21/1 -> Product6/1, Product2/2
  Constant1/1 -> Product6/2
  Product6/1 -> Product7/3
  Product7/1 -> Add2/1  "delta b"
  Add2/1 -> Product1/2, Scope1/1, To Workspace/1, Unit Delay1/1  "b(k)"

== system RWLNN_2m__/Subsystem3/Subsystem4 ==
  u(2) : Inport
  Gain : Gain  Gain=0.25
  Gain1 : Gain  Gain=-1
  Math Function : Math  SaturateOnIntegerOverflow=on
  Product1 : Product
  Product2 : Product
  Trigonometric Function : Trigonometry  Operator=cos
  O(2) = h(u(2)) : Outport
  wires:
  Product2/1 -> Gain1/1  "u(2) ^ 2"
  Product1/1 -> O(2) = h(u(2))/1
  Gain/1 -> Trigonometric Function/1  "0.25 * u(2)"
  Gain1/1 -> Math Function/1  "-(u(2) ^ 2)"
  Trigonometric Function/1 -> Product1/1
  u(2)/1 -> Product2/1, Product2/2, Gain/1
  Math Function/1 -> Product1/2

== system RWLNN_2m__/Subsystem3/Subsystem5 ==
  u(2) : Inport
  Gain : Gain  Gain=0.25
  Gain1 : Gain  Gain=-1
  Math Function : Math  SaturateOnIntegerOverflow=on
  Product1 : Product
  Product2 : Product
  Trigonometric Function : Trigonometry  Operator=cos
  O(2) = h(u(2)) : Outport
  wires:
  Math Function/1 -> Product1/2
  u(2)/1 -> Gain/1, Product2/2, Product2/1
  Trigonometric Function/1 -> Product1/1
  Gain1/1 -> Math Function/1  "-(u(2) ^ 2)"
  Gain/1 -> Trigonometric Function/1  "0.25 * u(2)"
  Product1/1 -> O(2) = h(u(2))/1
  Product2/1 -> Gain1/1  "u(2) ^ 2"

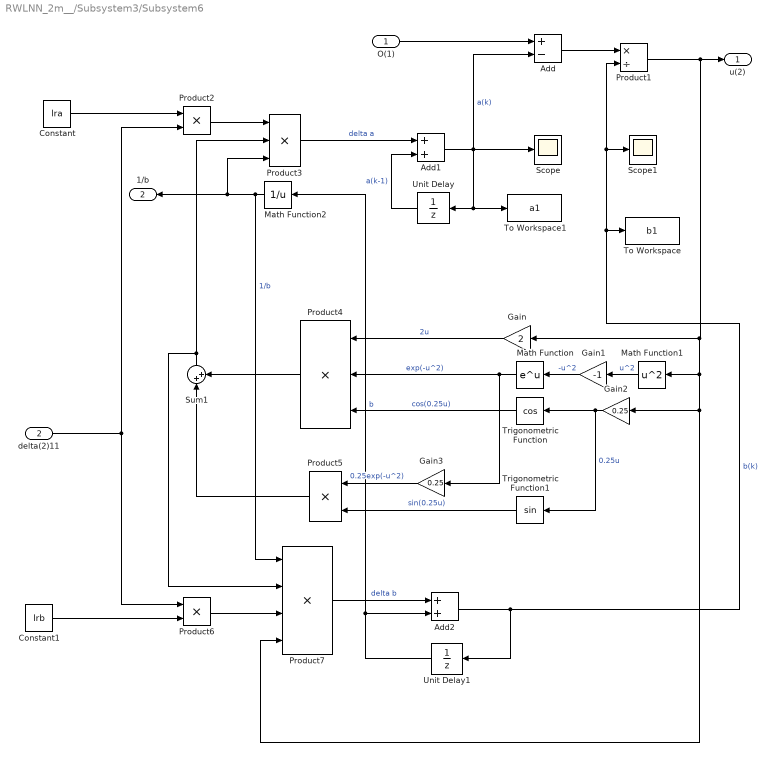
== system RWLNN_2m__/Subsystem3/Subsystem6 ==
  O(1) : Inport
  delta(2)11 : Inport  Port=2
  Add : Sum  Inputs=+-
  Add1 : Sum  Inputs=2
  Add2 : Sum  Inputs=2
  Constant : Constant  Value=lra
  Constant1 : Constant  Value=lrb
  Gain : Gain  Gain=2
  Gain1 : Gain  Gain=-1
  Gain2 : Gain  Gain=0.25
  Gain3 : Gain  Gain=0.25
  Math Function : Math  SaturateOnIntegerOverflow=on
  Math Function1 : Math  Operator=square  SaturateOnIntegerOverflow=on
  Math Function2 : Math  Operator=reciprocal  SaturateOnIntegerOverflow=on
  Product1 : Product  Inputs=*/
  Product2 : Product
  Product3 : Product  Inputs=3
  Product4 : Product  Inputs=3
  Product5 : Product
  Product6 : Product
  Product7 : Product  Inputs=4
  Scope : Scope
  Scope1 : Scope
  Sum1 : Sum  Inputs=|++
  To Workspace : ToWorkspace  VariableName=b1  SampleTime=-1
  To Workspace1 : ToWorkspace  VariableName=a1  SampleTime=-1
  Trigonometric Function : Trigonometry  Operator=cos
  Trigonometric Function1 : Trigonometry
  Unit Delay : UnitDelay  InitialCondition=-0.34  SampleTime=-1
  Unit Delay1 : UnitDelay  InitialCondition=0.56  SampleTime=-1
  u(2) : Outport
  1/b : Outport  Port=2
  wires:
  Add2/1 -> Unit Delay1/1, Product1/2, Scope1/1, To Workspace/1  "b(k)"
  Product7/1 -> Add2/1  "delta b"
  Product6/1 -> Product7/3
  Constant1/1 -> Product6/2
  delta(2)11/1 -> Product2/2, Product6/1
  Constant/1 -> Product2/1
  Unit Delay/1 -> Add1/2  "a(k-1)"
  Add1/1 -> Add/2, To Workspace1/1, Unit Delay/1, Scope/1  "a(k)"
  Product3/1 -> Add1/1  "delta a"
  Unit Delay1/1 -> Math Function2/1, Add2/2  "b"
  Math Function2/1 -> Product3/3, 1/b/1, Product7/1  "1/b"
  Sum1/1 -> Product7/2, Product3/2
  Product5/1 -> Sum1/1
  Trigonometric Function1/1 -> Product5/2  "sin(0.25u)"
  Gain3/1 -> Product5/1  "0.25exp(-u^2)"
  Product4/1 -> Sum1/2
  Trigonometric Function/1 -> Product4/3  "cos(0.25u)"
  Gain2/1 -> Trigonometric Function1/1, Trigonometric Function/1  "0.25u"
  Math Function/1 -> Gain3/1, Product4/2  "exp(-u^2)"
  Gain1/1 -> Math Function/1  "-u^2"
  Math Function1/1 -> Gain1/1  "u^2"
  Gain/1 -> Product4/1  "2u"
  Product1/1 -> u(2)/1, Gain/1, Math Function1/1, Gain2/1, Product7/4
  Product2/1 -> Product3/1
  Add/1 -> Product1/1
  O(1)/1 -> Add/1

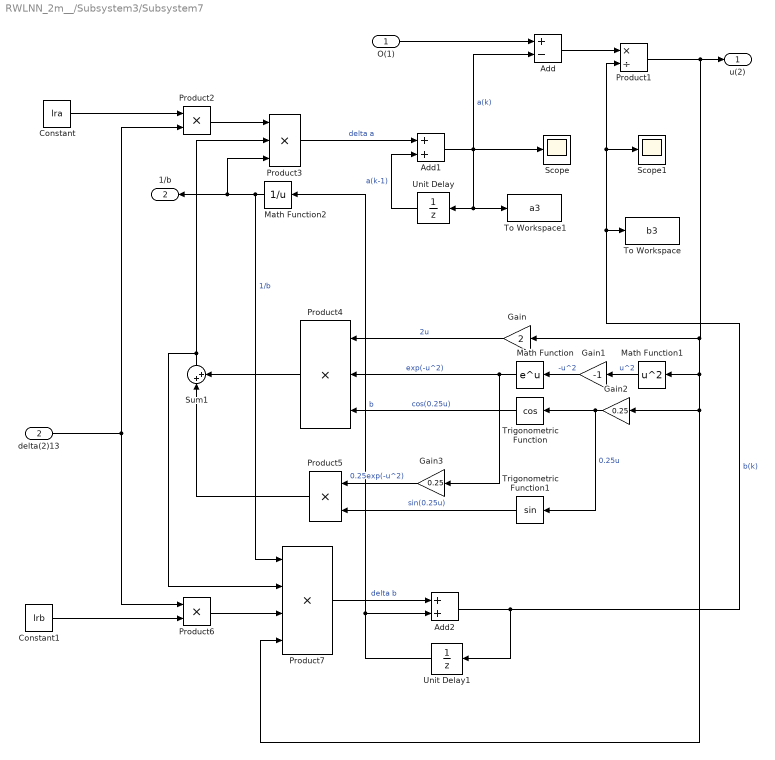
== system RWLNN_2m__/Subsystem3/Subsystem7 ==
  O(1) : Inport
  delta(2)13 : Inport  Port=2
  Add : Sum  Inputs=+-
  Add1 : Sum  Inputs=2
  Add2 : Sum  Inputs=2
  Constant : Constant  Value=lra
  Constant1 : Constant  Value=lrb
  Gain : Gain  Gain=2
  Gain1 : Gain  Gain=-1
  Gain2 : Gain  Gain=0.25
  Gain3 : Gain  Gain=0.25
  Math Function : Math  SaturateOnIntegerOverflow=on
  Math Function1 : Math  Operator=square  SaturateOnIntegerOverflow=on
  Math Function2 : Math  Operator=reciprocal  SaturateOnIntegerOverflow=on
  Product1 : Product  Inputs=*/
  Product2 : Product
  Product3 : Product  Inputs=3
  Product4 : Product  Inputs=3
  Product5 : Product
  Product6 : Product
  Product7 : Product  Inputs=4
  Scope : Scope
  Scope1 : Scope
  Sum1 : Sum  Inputs=|++
  To Workspace : ToWorkspace  VariableName=b3  SampleTime=-1
  To Workspace1 : ToWorkspace  VariableName=a3  SampleTime=-1
  Trigonometric Function : Trigonometry  Operator=cos
  Trigonometric Function1 : Trigonometry
  Unit Delay : UnitDelay  InitialCondition=0.36  SampleTime=-1
  Unit Delay1 : UnitDelay  InitialCondition=0.54  SampleTime=-1
  u(2) : Outport
  1/b : Outport  Port=2
  wires:
  Add2/1 -> Unit Delay1/1, Product1/2, Scope1/1, To Workspace/1  "b(k)"
  Product7/1 -> Add2/1  "delta b"
  Product6/1 -> Product7/3
  Constant1/1 -> Product6/2
  delta(2)13/1 -> Product2/2, Product6/1
  Constant/1 -> Product2/1
  Unit Delay/1 -> Add1/2  "a(k-1)"
  Add1/1 -> Add/2, To Workspace1/1, Unit Delay/1, Scope/1  "a(k)"
  Product3/1 -> Add1/1  "delta a"
  Unit Delay1/1 -> Math Function2/1, Add2/2  "b"
  Math Function2/1 -> 1/b/1, Product3/3, Product7/1  "1/b"
  Sum1/1 -> Product7/2, Product3/2
  Product5/1 -> Sum1/1
  Trigonometric Function1/1 -> Product5/2  "sin(0.25u)"
  Gain3/1 -> Product5/1  "0.25exp(-u^2)"
  Product4/1 -> Sum1/2
  Trigonometric Function/1 -> Product4/3  "cos(0.25u)"
  Gain2/1 -> Trigonometric Function1/1, Trigonometric Function/1  "0.25u"
  Math Function/1 -> Gain3/1, Product4/2  "exp(-u^2)"
  Gain1/1 -> Math Function/1  "-u^2"
  Math Function1/1 -> Gain1/1  "u^2"
  Gain/1 -> Product4/1  "2u"
  Product1/1 -> u(2)/1, Gain/1, Math Function1/1, Gain2/1, Product7/4
  Product2/1 -> Product3/1
  Add/1 -> Product1/1
  O(1)/1 -> Add/1

== system RWLNN_2m__/Subsystem3/Subsystem8 ==
  u(2) : Inport
  Gain : Gain  Gain=0.25
  Gain1 : Gain  Gain=-1
  Math Function : Math  SaturateOnIntegerOverflow=on
  Product1 : Product
  Product2 : Product
  Trigonometric Function : Trigonometry  Operator=cos
  O(2) = h(u(2)) : Outport
  wires:
  Math Function/1 -> Product1/2
  u(2)/1 -> Gain/1, Product2/2, Product2/1
  Trigonometric Function/1 -> Product1/1
  Gain1/1 -> Math Function/1  "-(u(2) ^ 2)"
  Gain/1 -> Trigonometric Function/1  "0.25 * u(2)"
  Product1/1 -> O(2) = h(u(2))/1
  Product2/1 -> Gain1/1  "u(2) ^ 2"

== system RWLNN_2m__/Subsystem3/Subsystem9 ==
  u(2) : Inport
  Gain : Gain  Gain=0.25
  Gain1 : Gain  Gain=-1
  Math Function : Math  SaturateOnIntegerOverflow=on
  Product1 : Product
  Product2 : Product
  Trigonometric Function : Trigonometry  Operator=cos
  O(2) = h(u(2)) : Outport
  wires:
  Product2/1 -> Gain1/1  "u(2) ^ 2"
  Product1/1 -> O(2) = h(u(2))/1
  Gain/1 -> Trigonometric Function/1  "0.25 * u(2)"
  Gain1/1 -> Math Function/1  "-(u(2) ^ 2)"
  Trigonometric Function/1 -> Product1/1
  u(2)/1 -> Product2/1, Product2/2, Gain/1
  Math Function/1 -> Product1/2
